simulink model "robot2"  (R2016a)
settings: Solver=FixedStepAuto  StartTime=0.0  StopTime=10.0  FixedStep=0.001  RelTol=1e-3
libraries: simulink x4
settings Model: Creator=Shinelon  LastModifiedBy=Shinelon

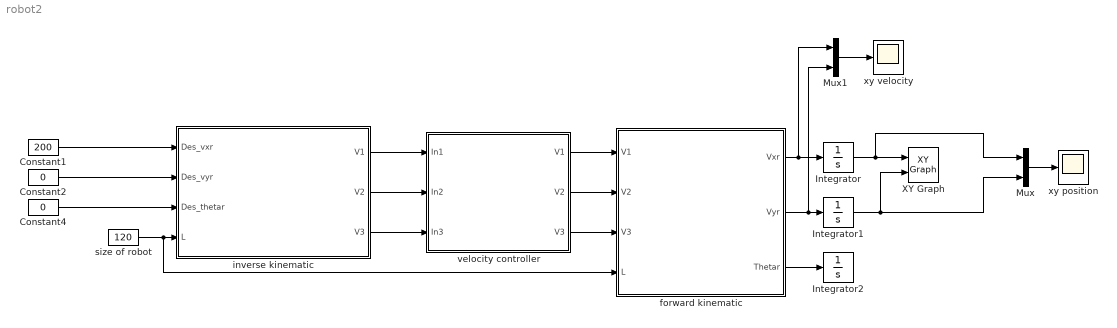
== system robot2 ==
  Constant1 : Constant  Value=200
  Constant2 : Constant  Value=0
  Constant4 : Constant  Value=0
  Integrator : Integrator
  Integrator1 : Integrator
  Integrator2 : Integrator
  Mux : Mux  Inputs=2
  Mux1 : Mux  Inputs=2
  XY Graph : simulink/Sinks/XY Graph  xmin=-1000  xmax=1000  ymin=-1000  ymax=1000  st=-1
  "forward kinematic " : MATLAB Function  TreatAsAtomicUnit=on
  "inverse kinematic " : MATLAB Function  TreatAsAtomicUnit=on
  "size of robot " : Constant  Value=120
  velocity controller : Subsystem
  "xy position " : Scope
  "xy velocity " : Scope
  wires:
  "size of robot "/1 -> "inverse kinematic "/4(L), "forward kinematic "/4(L)
  Constant4/1 -> "inverse kinematic "/3(Des_thetar)
  Constant2/1 -> "inverse kinematic "/2(Des_vyr)
  Constant1/1 -> "inverse kinematic "/1(Des_vxr)
  "forward kinematic "/1(Vxr) -> Mux1/1, Integrator/1
  Integrator/1 -> Mux/1, XY Graph/1
  "forward kinematic "/2(Vyr) -> Mux1/2, Integrator1/1
  Integrator1/1 -> Mux/2, XY Graph/2
  "forward kinematic "/3(Thetar) -> Integrator2/1
  "inverse kinematic "/1(V1) -> velocity controller/1(In1)
  "inverse kinematic "/2(V2) -> velocity controller/2(In2)
  "inverse kinematic "/3(V3) -> velocity controller/3(In3)
  velocity controller/1(V1) -> "forward kinematic "/1(V1)
  velocity controller/2(V2) -> "forward kinematic "/2(V2)
  velocity controller/3(V3) -> "forward kinematic "/3(V3)
  Mux/1 -> "xy position "/1
  Mux1/1 -> "xy velocity "/1

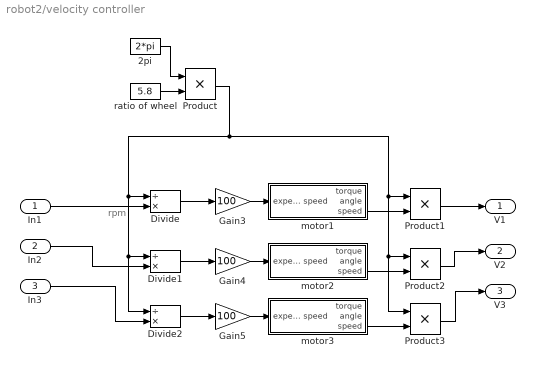
== system robot2/velocity controller ==
  note: rpm
  In1 : Inport
  In2 : Inport  Port=2
  In3 : Inport  Port=3
  2pi : Constant  Value=2*pi
  Divide : Product  Inputs=/*
  Divide1 : Product  Inputs=/*
  Divide2 : Product  Inputs=/*
  Gain3 : Gain  Gain=100
  Gain4 : Gain  Gain=100
  Gain5 : Gain  Gain=100
  Product{,1..3} (4 alike) : Product
  "motor1 " : Subsystem
  motor2 : Subsystem
  "motor3 " : Subsystem
  ratio of wheel : Constant  Value=5.8
  V1 : Outport
  V2 : Outport  Port=2
  V3 : Outport  Port=3
  wires:
  motor2/3("speed ") -> Product2/2
  Gain5/1 -> "motor3 "/1("expected speed ")
  Divide2/1 -> Gain5/1
  Divide1/1 -> Gain4/1
  Gain4/1 -> motor2/1("expected speed ")
  In1/1 -> Divide/2
  In2/1 -> Divide1/2
  Divide/1 -> Gain3/1
  In3/1 -> Divide2/2
  "motor3 "/3("speed ") -> Product3/2
  Product3/1 -> V3/1
  Product2/1 -> V2/1
  Gain3/1 -> "motor1 "/1("expected speed ")
  "motor1 "/3("speed ") -> Product1/2
  Product1/1 -> V1/1
  Product/1 -> Divide/1, Divide2/1, Divide1/1, Product3/1, Product2/1, Product1/1
  2pi/1 -> Product/1
  ratio of wheel/1 -> Product/2

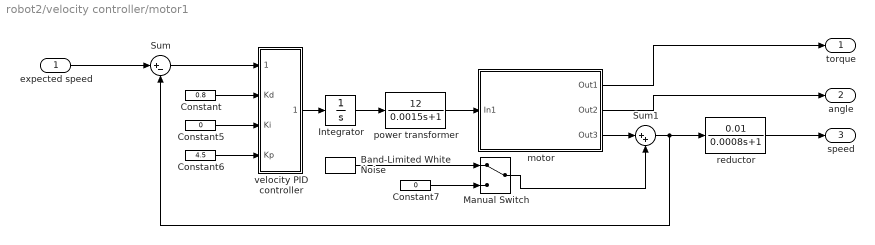
== system robot2/velocity controller/motor1  ==
  "expected speed " : Inport
  Band-Limited White Noise : simulink/Sources/Band-Limited White Noise  Cov=0.01  Ts=0.001  seed=[2331]
  Constant : Constant  Value=0.8
  Constant5 : Constant  Value=0
  Constant6 : Constant  Value=4.5
  Constant7 : Constant  Value=0
  Integrator : Integrator
  Manual Switch : ManualSwitch
  Sum : Sum  Inputs=|+-
  Sum1 : Sum  Inputs=|++
  "motor " : Subsystem  mask(DC motor subsystem){R=2, L=0.5, Km=0.1, Kf=0.2, Kemf=0.1, J=0.1}
      mask prompts: R "Resistor"; L "Inductor"; Km "Torque Constant"; Kf "Viscous Friction Constant"; Kemf "Back EMF Votage Constant"; J "Inertial Load"
      mask help:
      | This is a DC motor subsystem
      | Input : Control Signal
      | Output : Motor Rate
      mask init:
      | R=2;
      | L=0.5;
      | Km=0.1;
      | Kemf=0.1;
      | Kf=0.2;
      | J=0.02;
      mask Display:
      | color('red');port_label('input',1,'Control Signal');
      | color('red');port_label('output',1,'Torque');
      | color('red');port_label('output',2,'Angle');
      | color('red');port_label('output',3,'Speed');
      | image(imread('E:\matlab\simulink model\DC motor model\timg.jpg'))
  power transformer : TransferFcn  Numerator=[12]  Denominator=[0.0015 1]
  reductor : TransferFcn  Numerator=[0.01]  Denominator=[0.0008 1]
  "velocity PID controller " : Subsystem
  torque : Outport
  "angle " : Outport  Port=2
  "speed " : Outport  Port=3
  wires:
  Manual Switch/1 -> Sum1/2
  Sum/1 -> "velocity PID controller "/1(e(k))
  Constant/1 -> "velocity PID controller "/2("Kd ")
  Constant5/1 -> "velocity PID controller "/3("Ki ")
  Constant6/1 -> "velocity PID controller "/4("Kp ")
  Integrator/1 -> power transformer/1
  power transformer/1 -> "motor "/1(In1)
  Band-Limited White Noise/1 -> Manual Switch/1
  "velocity PID controller "/1(u(k)) -> Integrator/1
  reductor/1 -> "speed "/1
  "motor "/3(Out3) -> Sum1/1
  Sum1/1 -> reductor/1, Sum/2
  Constant7/1 -> Manual Switch/2
  "motor "/2(Out2) -> "angle "/1
  "motor "/1(Out1) -> torque/1
  "expected speed "/1 -> Sum/1

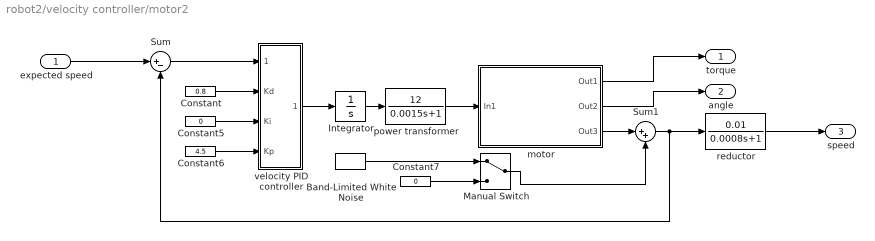
== system robot2/velocity controller/motor2 ==
  "expected speed " : Inport
  Band-Limited White Noise : simulink/Sources/Band-Limited White Noise  Cov=0.01  Ts=0.001  seed=[2341]
  Constant : Constant  Value=0.8
  Constant5 : Constant  Value=0
  Constant6 : Constant  Value=4.5
  Constant7 : Constant  Value=0
  Integrator : Integrator
  Manual Switch : ManualSwitch
  Sum : Sum  Inputs=|+-
  Sum1 : Sum  Inputs=|++
  "motor " : Subsystem  mask(DC motor subsystem){R=2, L=0.5, Km=0.1, Kf=0.2, Kemf=0.1, J=0.1}
      mask prompts: R "Resistor"; L "Inductor"; Km "Torque Constant"; Kf "Viscous Friction Constant"; Kemf "Back EMF Votage Constant"; J "Inertial Load"
      mask help:
      | This is a DC motor subsystem
      | Input : Control Signal
      | Output : Motor Rate
      mask init:
      | R=2;
      | L=0.5;
      | Km=0.1;
      | Kemf=0.1;
      | Kf=0.2;
      | J=0.02;
      mask Display:
      | color('red');port_label('input',1,'Control Signal');
      | color('red');port_label('output',1,'Torque');
      | color('red');port_label('output',2,'Angle');
      | color('red');port_label('output',3,'Speed');
      | image(imread('E:\matlab\simulink model\DC motor model\timg.jpg'))
  power transformer : TransferFcn  Numerator=[12]  Denominator=[0.0015 1]
  reductor : TransferFcn  Numerator=[0.01]  Denominator=[0.0008 1]
  "velocity PID controller " : Subsystem
  torque : Outport
  "angle " : Outport  Port=2
  "speed " : Outport  Port=3
  wires:
  Manual Switch/1 -> Sum1/2
  Sum/1 -> "velocity PID controller "/1(e(k))
  Constant/1 -> "velocity PID controller "/2("Kd ")
  Constant5/1 -> "velocity PID controller "/3("Ki ")
  Constant6/1 -> "velocity PID controller "/4("Kp ")
  Integrator/1 -> power transformer/1
  power transformer/1 -> "motor "/1(In1)
  Band-Limited White Noise/1 -> Manual Switch/1
  "velocity PID controller "/1(u(k)) -> Integrator/1
  reductor/1 -> "speed "/1
  "motor "/3(Out3) -> Sum1/1
  Sum1/1 -> reductor/1, Sum/2
  Constant7/1 -> Manual Switch/2
  "motor "/2(Out2) -> "angle "/1
  "motor "/1(Out1) -> torque/1
  "expected speed "/1 -> Sum/1

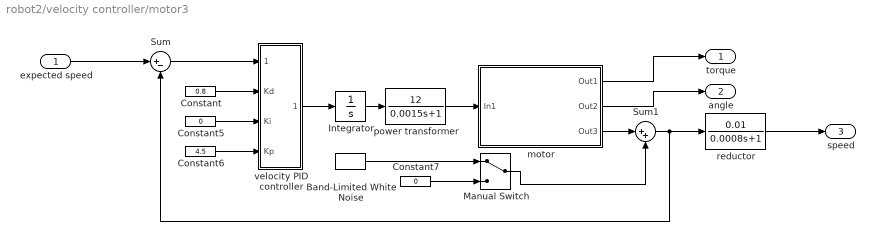
== system robot2/velocity controller/motor3  ==
  "expected speed " : Inport
  Band-Limited White Noise : simulink/Sources/Band-Limited White Noise  Cov=0.01  Ts=0.001  seed=[23341]
  Constant : Constant  Value=0.8
  Constant5 : Constant  Value=0
  Constant6 : Constant  Value=4.5
  Constant7 : Constant  Value=0
  Integrator : Integrator
  Manual Switch : ManualSwitch
  Sum : Sum  Inputs=|+-
  Sum1 : Sum  Inputs=|++
  "motor " : Subsystem  mask(DC motor subsystem){R=2, L=0.5, Km=0.1, Kf=0.2, Kemf=0.1, J=0.1}
      mask prompts: R "Resistor"; L "Inductor"; Km "Torque Constant"; Kf "Viscous Friction Constant"; Kemf "Back EMF Votage Constant"; J "Inertial Load"
      mask help:
      | This is a DC motor subsystem
      | Input : Control Signal
      | Output : Motor Rate
      mask init:
      | R=2;
      | L=0.5;
      | Km=0.1;
      | Kemf=0.1;
      | Kf=0.2;
      | J=0.02;
      mask Display:
      | color('red');port_label('input',1,'Control Signal');
      | color('red');port_label('output',1,'Torque');
      | color('red');port_label('output',2,'Angle');
      | color('red');port_label('output',3,'Speed');
      | image(imread('E:\matlab\simulink model\DC motor model\timg.jpg'))
  power transformer : TransferFcn  Numerator=[12]  Denominator=[0.0015 1]
  reductor : TransferFcn  Numerator=[0.01]  Denominator=[0.0008 1]
  "velocity PID controller " : Subsystem
  torque : Outport
  "angle " : Outport  Port=2
  "speed " : Outport  Port=3
  wires:
  Manual Switch/1 -> Sum1/2
  Sum/1 -> "velocity PID controller "/1(e(k))
  Constant/1 -> "velocity PID controller "/2("Kd ")
  Constant5/1 -> "velocity PID controller "/3("Ki ")
  Constant6/1 -> "velocity PID controller "/4("Kp ")
  Integrator/1 -> power transformer/1
  power transformer/1 -> "motor "/1(In1)
  Band-Limited White Noise/1 -> Manual Switch/1
  "velocity PID controller "/1(u(k)) -> Integrator/1
  reductor/1 -> "speed "/1
  "motor "/3(Out3) -> Sum1/1
  Sum1/1 -> reductor/1, Sum/2
  Constant7/1 -> Manual Switch/2
  "motor "/2(Out2) -> "angle "/1
  "motor "/1(Out1) -> torque/1
  "expected speed "/1 -> Sum/1

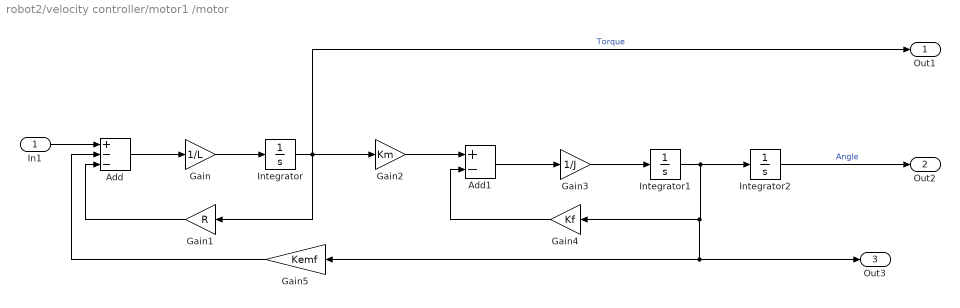
== system robot2/velocity controller/motor1 /motor  ==
  In1 : Inport
  Add : Sum  Inputs=+--
  Add1 : Sum  Inputs=+-
  Gain : Gain  Gain=1/L
  Gain1 : Gain  Gain=R
  Gain2 : Gain  Gain=Km
  Gain3 : Gain  Gain=1/J
  Gain4 : Gain  Gain=Kf
  Gain5 : Gain  Gain=Kemf
  Integrator : Integrator
  Integrator1 : Integrator
  Integrator2 : Integrator
  Out1 : Outport
  Out2 : Outport  Port=2
  Out3 : Outport  Port=3
  wires:
  Gain5/1 -> Add/2
  Integrator/1 -> Out1/1, Gain2/1, Gain1/1  "Torque"
  Integrator2/1 -> Out2/1  "Angle"
  Add/1 -> Gain/1
  Gain/1 -> Integrator/1
  Gain1/1 -> Add/3
  Gain2/1 -> Add1/1
  Add1/1 -> Gain3/1
  Gain3/1 -> Integrator1/1
  Integrator1/1 -> Integrator2/1, Out3/1, Gain5/1, Gain4/1
  Gain4/1 -> Add1/2
  In1/1 -> Add/1

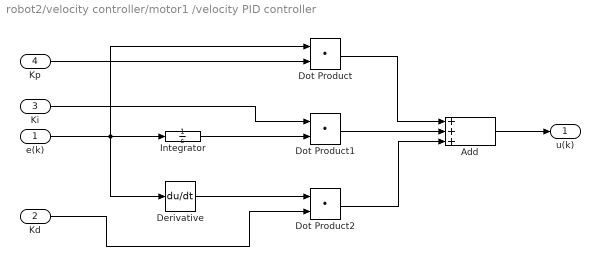
== system robot2/velocity controller/motor1 /velocity PID controller  ==
  e(k) : Inport
  "Kd " : Inport  Port=2
  "Ki " : Inport  Port=3
  "Kp " : Inport  Port=4
  Add : Sum  Inputs=+++
  Derivative : Derivative
  Dot Product : DotProduct  InputSameDT=on  OutDataTypeStr=Inherit: Inherit via internal rule
  Dot Product1 : DotProduct  InputSameDT=on  OutDataTypeStr=Inherit: Inherit via internal rule
  Dot Product2 : DotProduct  InputSameDT=on  OutDataTypeStr=Inherit: Inherit via internal rule
  Integrator : Integrator
  u(k) : Outport
  wires:
  "Ki "/1 -> Dot Product1/1
  "Kp "/1 -> Dot Product/2
  Add/1 -> u(k)/1
  Derivative/1 -> Dot Product2/1
  Dot Product/1 -> Add/1
  Dot Product2/1 -> Add/3
  Integrator/1 -> Dot Product1/2
  "Kd "/1 -> Dot Product2/2
  Dot Product1/1 -> Add/2
  e(k)/1 -> Dot Product/1, Integrator/1, Derivative/1

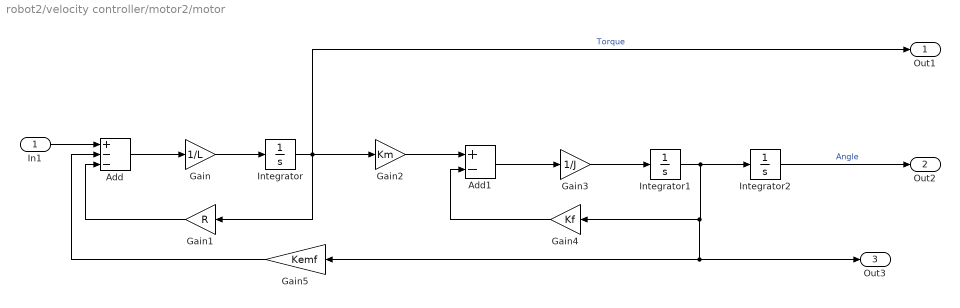
== system robot2/velocity controller/motor2/motor  ==
  In1 : Inport
  Add : Sum  Inputs=+--
  Add1 : Sum  Inputs=+-
  Gain : Gain  Gain=1/L
  Gain1 : Gain  Gain=R
  Gain2 : Gain  Gain=Km
  Gain3 : Gain  Gain=1/J
  Gain4 : Gain  Gain=Kf
  Gain5 : Gain  Gain=Kemf
  Integrator : Integrator
  Integrator1 : Integrator
  Integrator2 : Integrator
  Out1 : Outport
  Out2 : Outport  Port=2
  Out3 : Outport  Port=3
  wires:
  Gain5/1 -> Add/2
  Integrator/1 -> Out1/1, Gain2/1, Gain1/1  "Torque"
  Integrator2/1 -> Out2/1  "Angle"
  Add/1 -> Gain/1
  Gain/1 -> Integrator/1
  Gain1/1 -> Add/3
  Gain2/1 -> Add1/1
  Add1/1 -> Gain3/1
  Gain3/1 -> Integrator1/1
  Integrator1/1 -> Integrator2/1, Out3/1, Gain5/1, Gain4/1
  Gain4/1 -> Add1/2
  In1/1 -> Add/1

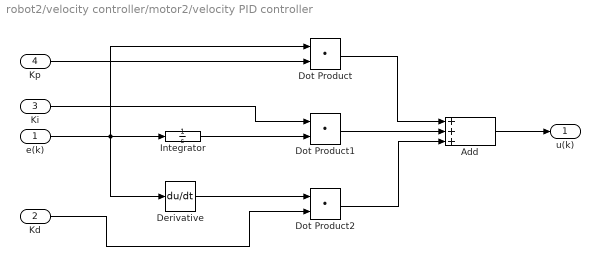
== system robot2/velocity controller/motor2/velocity PID controller  ==
  e(k) : Inport
  "Kd " : Inport  Port=2
  "Ki " : Inport  Port=3
  "Kp " : Inport  Port=4
  Add : Sum  Inputs=+++
  Derivative : Derivative
  Dot Product : DotProduct  InputSameDT=on  OutDataTypeStr=Inherit: Inherit via internal rule
  Dot Product1 : DotProduct  InputSameDT=on  OutDataTypeStr=Inherit: Inherit via internal rule
  Dot Product2 : DotProduct  InputSameDT=on  OutDataTypeStr=Inherit: Inherit via internal rule
  Integrator : Integrator
  u(k) : Outport
  wires:
  "Ki "/1 -> Dot Product1/1
  "Kp "/1 -> Dot Product/2
  Add/1 -> u(k)/1
  Derivative/1 -> Dot Product2/1
  Dot Product/1 -> Add/1
  Dot Product2/1 -> Add/3
  Integrator/1 -> Dot Product1/2
  "Kd "/1 -> Dot Product2/2
  Dot Product1/1 -> Add/2
  e(k)/1 -> Dot Product/1, Integrator/1, Derivative/1

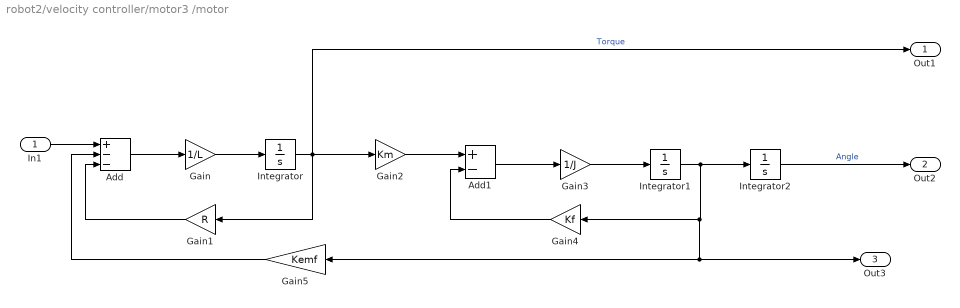
== system robot2/velocity controller/motor3 /motor  ==
  In1 : Inport
  Add : Sum  Inputs=+--
  Add1 : Sum  Inputs=+-
  Gain : Gain  Gain=1/L
  Gain1 : Gain  Gain=R
  Gain2 : Gain  Gain=Km
  Gain3 : Gain  Gain=1/J
  Gain4 : Gain  Gain=Kf
  Gain5 : Gain  Gain=Kemf
  Integrator : Integrator
  Integrator1 : Integrator
  Integrator2 : Integrator
  Out1 : Outport
  Out2 : Outport  Port=2
  Out3 : Outport  Port=3
  wires:
  Gain5/1 -> Add/2
  Integrator/1 -> Out1/1, Gain2/1, Gain1/1  "Torque"
  Integrator2/1 -> Out2/1  "Angle"
  Add/1 -> Gain/1
  Gain/1 -> Integrator/1
  Gain1/1 -> Add/3
  Gain2/1 -> Add1/1
  Add1/1 -> Gain3/1
  Gain3/1 -> Integrator1/1
  Integrator1/1 -> Integrator2/1, Out3/1, Gain5/1, Gain4/1
  Gain4/1 -> Add1/2
  In1/1 -> Add/1

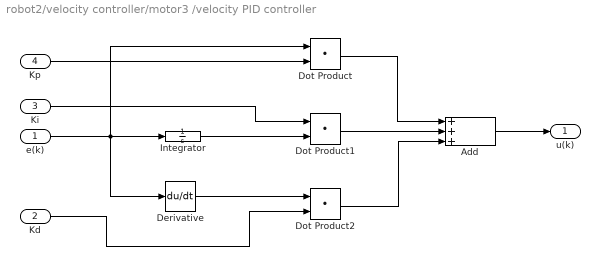
== system robot2/velocity controller/motor3 /velocity PID controller  ==
  e(k) : Inport
  "Kd " : Inport  Port=2
  "Ki " : Inport  Port=3
  "Kp " : Inport  Port=4
  Add : Sum  Inputs=+++
  Derivative : Derivative
  Dot Product : DotProduct  InputSameDT=on  OutDataTypeStr=Inherit: Inherit via internal rule
  Dot Product1 : DotProduct  InputSameDT=on  OutDataTypeStr=Inherit: Inherit via internal rule
  Dot Product2 : DotProduct  InputSameDT=on  OutDataTypeStr=Inherit: Inherit via internal rule
  Integrator : Integrator
  u(k) : Outport
  wires:
  "Ki "/1 -> Dot Product1/1
  "Kp "/1 -> Dot Product/2
  Add/1 -> u(k)/1
  Derivative/1 -> Dot Product2/1
  Dot Product/1 -> Add/1
  Dot Product2/1 -> Add/3
  Integrator/1 -> Dot Product1/2
  "Kd "/1 -> Dot Product2/2
  Dot Product1/1 -> Add/2
  e(k)/1 -> Dot Product/1, Integrator/1, Derivative/1

== matlab function robot2/inverse kinematic  ==
  data: Des_vxr input; V1 output; Des_vyr input; Des_thetar input; V2 output; V3 output; L input
function [V1,V2,V3] = inverse_kinematic(Des_vxr,Des_vyr,Des_thetar,L)

transfer_matrix = [cos(1/6*pi) cos(5/6*pi) cos(3/2*pi);
                   sin(1/6*pi) sin(5/6*pi) sin(3/2*pi);
                   1/(3*L)   1/(3*L)  1/(3*L) ];

inverse_model = inv(transfer_matrix);

%result = [Des_vxr,Des_vyr,Des_thetar]'/transfer_matrix;
result = inverse_model*[Des_vxr,Des_vyr,Des_thetar]';

V1 = result(1);
V2 = result(2);
V3 = result(3);

== matlab function robot2/forward kinematic  ==
  data: V1 input; Vxr output; V2 input; V3 input; Vyr output; Thetar output; L input
function [Vxr,Vyr,Thetar] = forward_kinematic(V1,V2,V3,L)

%   L is distance between center and middle of wheel



transfer_matrix = [cos(1/6*pi) cos(5/6*pi) cos(3/2*pi);
                   sin(1/6*pi) sin(5/6*pi) sin(3/2*pi);
                   1/(3*L)   1/(3*L)  1/(3*L) ];
result = transfer_matrix*[V1,V2,V3]';

Vxr = result(1);
Vyr = result(2);
Thetar = result(3);
